simulink model "svpwm_equilibrado"  (R2022b)
settings: Solver=VariableStepAuto  StartTime=0.0  StopTime=0.02  MaxStep=0.00001  RelTol=1e-3
libraries: eeStairGenerator x1
settings Model: Creator=ramuj  LastModifiedBy=ramuj
settings DebuggingCC: UnconnectedInputMsg=warning  UnconnectedOutputMsg=warning  UnconnectedLineMsg=warning
settings ModelReferenceCC: EnableRefExpFcnMdlSchedulingChecks=on
settings RTWCC: DLArmComputeVersion=19.05

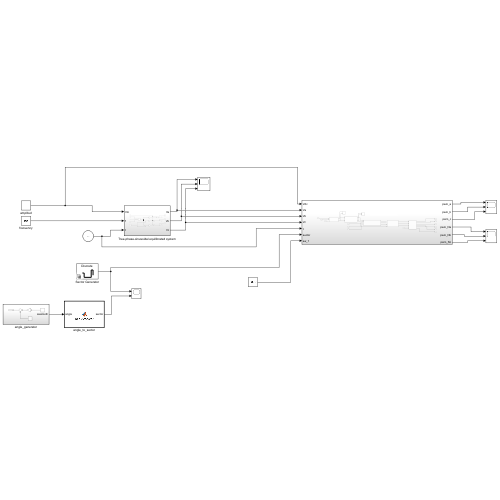
[thumbnail: Simulink's stored preview of the top-level diagram]
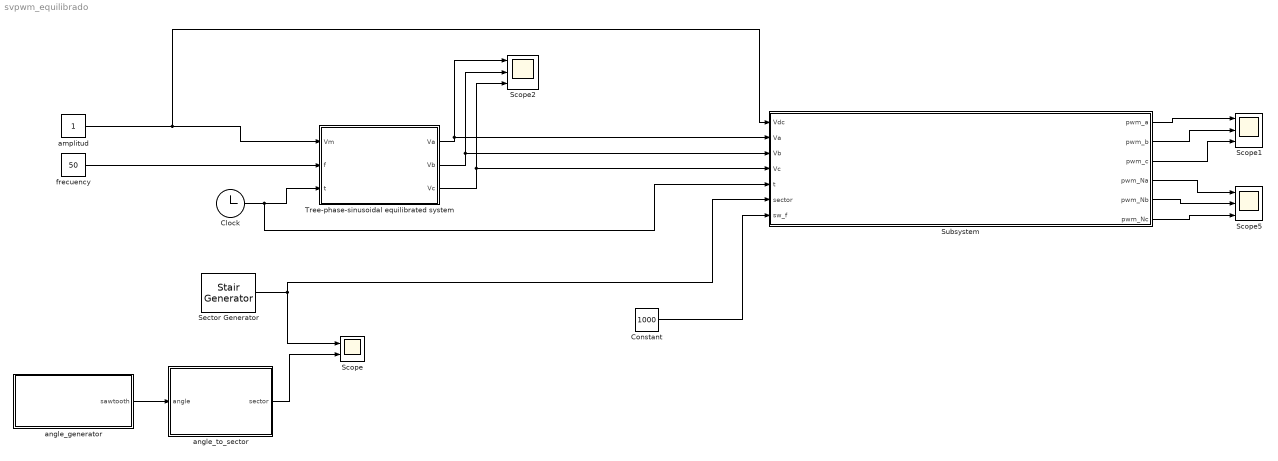
== system svpwm_equilibrado ==
  Clock : Clock
  Constant : Constant  Value=1000
  Scope : Scope  NumInputPorts=2
  Scope1 : Scope  NumInputPorts=3
  Scope2 : Scope  NumInputPorts=3
  Scope5 : Scope  NumInputPorts=3
  Sector Generator : eeStairGenerator/Stair Generator  LabelModeActiveChoice=Discrete  TimeInput=(0.02/6)*[0 1 2 3 4 5 6]  AmplitudeInput=[1 2 3 4 5 6 1]  SampleTime=(0.02/6)/10  RepeatPattern=off  OutDataTypeStr=double
      settings: LibrarySourceBlock=ee_sl_lib/General Control/Stair Generator
  Subsystem : Subsystem
  Tree-phase-sinusoidal equilibrated system : Subsystem
  amplitud : Constant
  angle_generator : Subsystem
  angle_to_sector : MATLAB Function  TreatAsAtomicUnit=on
  frecuency : Constant  Value=50
  wires:
  Tree-phase-sinusoidal equilibrated system/1(Va) -> Scope2/1, Subsystem/2(Va)
  Tree-phase-sinusoidal equilibrated system/2(Vb) -> Scope2/2, Subsystem/3(Vb)
  Tree-phase-sinusoidal equilibrated system/3(Vc) -> Scope2/3, Subsystem/4(Vc)
  Clock/1 -> Subsystem/5(t), Tree-phase-sinusoidal equilibrated system/3(t)
  frecuency/1 -> Tree-phase-sinusoidal equilibrated system/2(f)
  amplitud/1 -> Subsystem/1(Vdc), Tree-phase-sinusoidal equilibrated system/1(Vm)
  Sector Generator/1 -> Subsystem/6(sector), Scope/1
  Subsystem/1(pwm_a) -> Scope1/1
  Subsystem/2(pwm_b) -> Scope1/2
  Subsystem/3(pwm_c) -> Scope1/3
  Subsystem/4(pwm_Na) -> Scope5/1
  Subsystem/5(pwm_Nb) -> Scope5/2
  Subsystem/6(pwm_Nc) -> Scope5/3
  Constant/1 -> Subsystem/7(sw_f)
  angle_to_sector/1(sector) -> Scope/2
  angle_generator/1(sawtooth) -> angle_to_sector/1(angle)

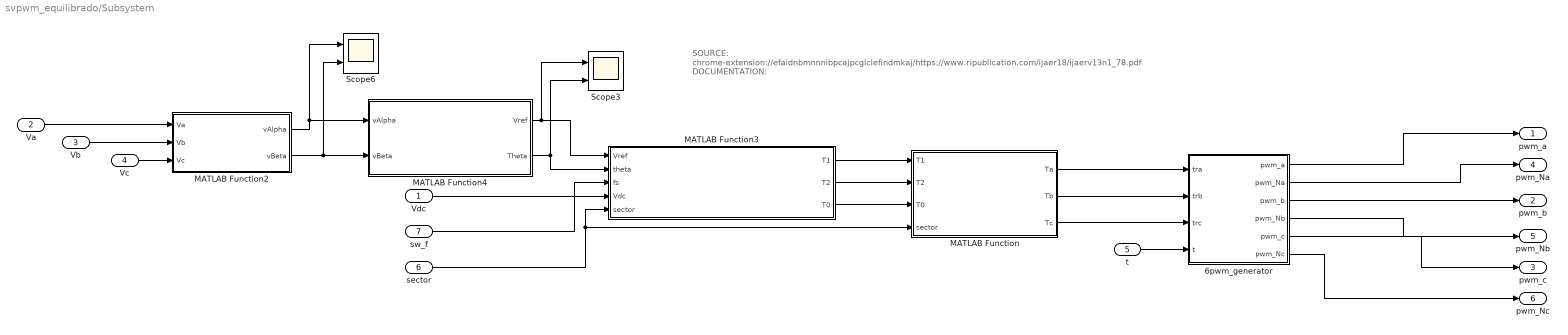
== system svpwm_equilibrado/Subsystem ==
  note: SOURCE:
      | chrome-extension://efaidnbmnnnibpcajpcglclefindmkaj/https://www.ripublication.com/ijaer18/ijaerv13n1_78.pdf
      | DOCUMENTATION:
  Vdc : Inport
  Va : Inport  Port=2
  Vb : Inport  Port=3
  Vc : Inport  Port=4
  t : Inport  Port=5
  sector : Inport  Port=6
  sw_f : Inport  Port=7
  6pwm_generator : Subsystem
  MATLAB Function : MATLAB Function  TreatAsAtomicUnit=on
  MATLAB Function2 : MATLAB Function  TreatAsAtomicUnit=on
  MATLAB Function3 : MATLAB Function  TreatAsAtomicUnit=on
  MATLAB Function4 : MATLAB Function  TreatAsAtomicUnit=on
  Scope3 : Scope  NumInputPorts=2
  Scope6 : Scope  NumInputPorts=2
  pwm_a : Outport
  pwm_b : Outport  Port=2
  pwm_c : Outport  Port=3
  pwm_Na : Outport  Port=4
  pwm_Nb : Outport  Port=5
  pwm_Nc : Outport  Port=6
  wires:
  sector/1 -> MATLAB Function3/5(sector), MATLAB Function/4(sector)
  MATLAB Function3/1(T1) -> MATLAB Function/1(T1)
  MATLAB Function2/2(vBeta) -> MATLAB Function4/2(vBeta), Scope6/2
  MATLAB Function4/2(Theta) -> Scope3/2, MATLAB Function3/2(theta)
  MATLAB Function4/1(Vref) -> MATLAB Function3/1(Vref), Scope3/1
  MATLAB Function3/3(T0) -> MATLAB Function/3(T0)
  MATLAB Function3/2(T2) -> MATLAB Function/2(T2)
  6pwm_generator/6(pwm_Nc) -> pwm_Nc/1
  Vdc/1 -> MATLAB Function3/4(Vdc)
  MATLAB Function2/1(vAlpha) -> MATLAB Function4/1(vAlpha), Scope6/1
  MATLAB Function/2(Tb) -> 6pwm_generator/2(trb)
  6pwm_generator/2(pwm_Na) -> pwm_Na/1
  6pwm_generator/5(pwm_c) -> pwm_c/1
  MATLAB Function/1(Ta) -> 6pwm_generator/1(tra)
  sw_f/1 -> MATLAB Function3/3(fs)
  MATLAB Function/3(Tc) -> 6pwm_generator/3(trc)
  Vb/1 -> MATLAB Function2/2(Vb)
  Va/1 -> MATLAB Function2/1(Va)
  Vc/1 -> MATLAB Function2/3(Vc)
  t/1 -> 6pwm_generator/4(t)
  6pwm_generator/1(pwm_a) -> pwm_a/1
  6pwm_generator/3(pwm_b) -> pwm_b/1
  6pwm_generator/4(pwm_Nb) -> pwm_Nb/1

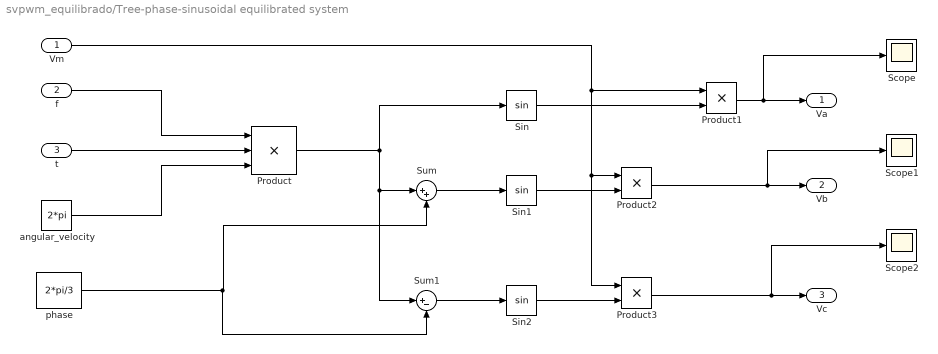
== system svpwm_equilibrado/Tree-phase-sinusoidal equilibrated system ==
  Vm : Inport
  f : Inport  Port=2
  t : Inport  Port=3
  Product : Product  Inputs=3
  Product1 : Product
  Product2 : Product
  Product3 : Product
  Scope : Scope
  Scope1 : Scope
  Scope2 : Scope
  Sin : Trigonometry
  Sin1 : Trigonometry
  Sin2 : Trigonometry
  Sum : Sum  Inputs=|++
  Sum1 : Sum  Inputs=|+-
  angular_velocity : Constant  Value=2*pi
  phase : Constant  Value=2*pi/3
  Va : Outport
  Vb : Outport  Port=2
  Vc : Outport  Port=3
  wires:
  f/1 -> Product/1
  t/1 -> Product/2
  angular_velocity/1 -> Product/3
  Product/1 -> Sin/1, Sum/1, Sum1/1
  Vm/1 -> Product3/1, Product2/1, Product1/1
  Sin/1 -> Product1/2
  Product1/1 -> Scope/1, Va/1
  phase/1 -> Sum1/2, Sum/2
  Sum/1 -> Sin1/1
  Sin1/1 -> Product2/2
  Product2/1 -> Scope1/1, Vb/1
  Sum1/1 -> Sin2/1
  Sin2/1 -> Product3/2
  Product3/1 -> Scope2/1, Vc/1

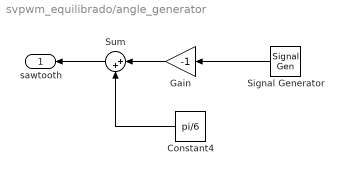
== system svpwm_equilibrado/angle_generator ==
  Constant4 : Constant  Value=pi/6
  Gain : Gain  Gain=-1
  Signal Generator : SignalGenerator  WaveForm=sawtooth  Amplitude=pi/6  Frequency=0.003  Units=rad/sec
  Sum : Sum  Inputs=|++
  sawtooth : Outport
  wires:
  Gain/1 -> Sum/1
  Constant4/1 -> Sum/2
  Signal Generator/1 -> Gain/1
  Sum/1 -> sawtooth/1

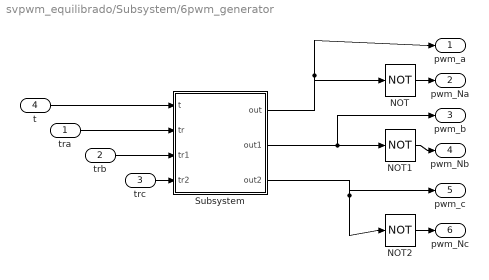
== system svpwm_equilibrado/Subsystem/6pwm_generator ==
  tra : Inport
  trb : Inport  Port=2
  trc : Inport  Port=3
  t : Inport  Port=4
  NOT : Logic  Operator=NOT  IconShape=distinctive  AllPortsSameDT=off  OutDataTypeStr=boolean
  NOT1 : Logic  Operator=NOT  IconShape=distinctive  AllPortsSameDT=off  OutDataTypeStr=boolean
  NOT2 : Logic  Operator=NOT  IconShape=distinctive  AllPortsSameDT=off  OutDataTypeStr=boolean
  Subsystem : Subsystem
  pwm_a : Outport
  pwm_Na : Outport  Port=2
  pwm_b : Outport  Port=3
  pwm_Nb : Outport  Port=4
  pwm_c : Outport  Port=5
  pwm_Nc : Outport  Port=6
  wires:
  Subsystem/2(out1) -> NOT1/1, pwm_b/1
  Subsystem/3(out2) -> NOT2/1, pwm_c/1
  NOT1/1 -> pwm_Nb/1
  Subsystem/1(out) -> NOT/1, pwm_a/1
  tra/1 -> Subsystem/2(tr)
  NOT2/1 -> pwm_Nc/1
  trc/1 -> Subsystem/4(tr2)
  trb/1 -> Subsystem/3(tr1)
  t/1 -> Subsystem/1(t)
  NOT/1 -> pwm_Na/1

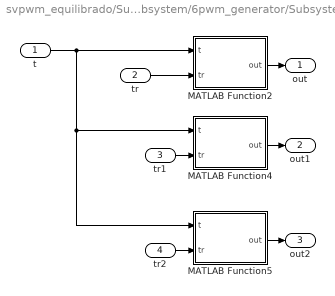
== system svpwm_equilibrado/Subsystem/6pwm_generator/Subsystem ==
  t : Inport
  tr : Inport  Port=2
  tr1 : Inport  Port=3
  tr2 : Inport  Port=4
  MATLAB Function2 : MATLAB Function  TreatAsAtomicUnit=on
  MATLAB Function4 : MATLAB Function  TreatAsAtomicUnit=on
  MATLAB Function5 : MATLAB Function  TreatAsAtomicUnit=on
  out : Outport
  out1 : Outport  Port=2
  out2 : Outport  Port=3
  wires:
  MATLAB Function4/1(out) -> out1/1
  tr2/1 -> MATLAB Function5/2(tr)
  tr1/1 -> MATLAB Function4/2(tr)
  tr/1 -> MATLAB Function2/2(tr)
  MATLAB Function2/1(out) -> out/1
  t/1 -> MATLAB Function5/1(t), MATLAB Function4/1(t), MATLAB Function2/1(t)
  MATLAB Function5/1(out) -> out2/1

== matlab function svpwm_equilibrado/Subsystem/MATLAB Function ==
  data: T1 input; T2 input; T0 input; Ta output; sector input; Tb output; Tc output
function [Ta, Tb, Tc] = switches(T1, T2, T0, sector)
switch sector
    case 1
        Ta = T1 + T2 + T0/2
        Tb = T2 + T0/2
        Tc = T0/2
    case 2
        Ta = T1 + T0/2
        Tb = T1 + T2 + T0/2
        Tc = T0/2
    case 3
        Ta = T0/2
        Tb = T1 + T2 + T0/2
        Tc = T2 + T0/2
    case 4
        Ta = T0/2
        Tb = T1 + T0/2
        Tc = T1 + T2 + T0/2
    case 5
        Ta = T2 + T0/2
        Tb = T0/2
        Tc = T1 + T2 + T0/2
    case 6
        Ta = T1 + T2 + T0/2
        Tb = T0/2
        Tc = T1 + T0/2
    otherwise
        Ta = 0
        Tb = 0
        Tc = 0
end

== matlab function svpwm_equilibrado/angle_to_sector ==
  data: angle input; sector output
function sector = angle2sector(angle)

angle = angle * (180/pi)

if angle > 0 & angle <= 60
    sector = 1
end
if angle > 60 & angle <= 120
    sector = 2
end
if angle > 120 & angle <= 180
    sector = 3
end
if angle > -180 & angle <= -120
    sector = 4
end
if angle > -120 & angle <= -60
    sector = 5
end
if angle > -60 & angle <= 0
    sector = 6
else
    sector = 0
end

== matlab function svpwm_equilibrado/Subsystem/MATLAB Function3 ==
  data: Vref input; T1 output; theta input; T2 output; T0 output; fs input; Vdc input; sector input
function [T1, T2, T0] = times(Vref, theta, fs, Vdc, sector)
Ts = 1/fs
T1 = (sqrt(3)*Ts*abs(Vref))/Vdc * sin((sector/3)*pi-theta)
T2 = (sqrt(3)*Ts*abs(Vref))/Vdc * sin(theta - ((sector-1)/3)*pi)
T0 = Ts - (T1 + T2)

== matlab function svpwm_equilibrado/Subsystem/6pwm_generator/Subsystem/MATLAB Function2 ==
  data: t input; out output; tr input
function out = pwm(t,tr)
if t>=tr
    out = 1
else 
    out = 0
end

== matlab function svpwm_equilibrado/Subsystem/6pwm_generator/Subsystem/MATLAB Function4 ==
  data: t input; out output; tr input
function out = pwm(t,tr)
if t>=tr
    out = 1
else 
    out = 0
end

== matlab function svpwm_equilibrado/Subsystem/6pwm_generator/Subsystem/MATLAB Function5 ==
  data: t input; out output; tr input
function out = pwm(t,tr)
if t>=tr
    out = 1
else 
    out = 0
end

== matlab function svpwm_equilibrado/Subsystem/MATLAB Function2 ==
  data: Va input; vAlpha output; Vb input; vBeta output; Vc input
function [vAlpha,vBeta] = alpha_beta(Va, Vb, Vc)
vAlpha = (2/3)*Va - (1/3)*Vb - (1/3)*Vc;
vBeta = (sqrt(3)/3)*Vb - (sqrt(3)/3)*Vc;

== matlab function svpwm_equilibrado/Subsystem/MATLAB Function4 ==
  data: vAlpha input; Vref output; vBeta input; Theta output
function [Vref,Theta] = generate_vref_theta(vAlpha, vBeta)
  Vref = sqrt((vAlpha^2) + (vBeta^2));
  Theta = atan2(vBeta, vAlpha);
